simulink model "main_simulink"  (R2019b)
settings: Solver=FixedStepAuto  StartTime=0.0  StopTime=2.5  FixedStep=0.01  RelTol=1e-3
values from neighbouring files (symbols this model uses):
  b = 0.1    [main.m]
  g = 9.8    [main.m]
  I = 0.006    [main.m]
  l = 0.3    [main.m]
  m = length(x)    [PRBS.m]    (also in gaplotbestindivg.m = sum(x) ./ n; main.m = 0.2)
  M = 0.5    [main.m]
libraries: simulink x1
settings Model: Creator=sansh  LastModifiedBy=rifky
settings DataIOCC: ReturnWorkspaceOutputs=off
settings DebuggingCC: ArithmeticOperatorsInVariantConditions=warning
settings SFSimCC: SimUseLocalCustomCode=off  CustomCodeUndefinedFunction=UseInterfaceOnly
settings RTWCC: RTWUseLocalCustomCode=off
settings CodeAppCC: StateflowObjectComments=on

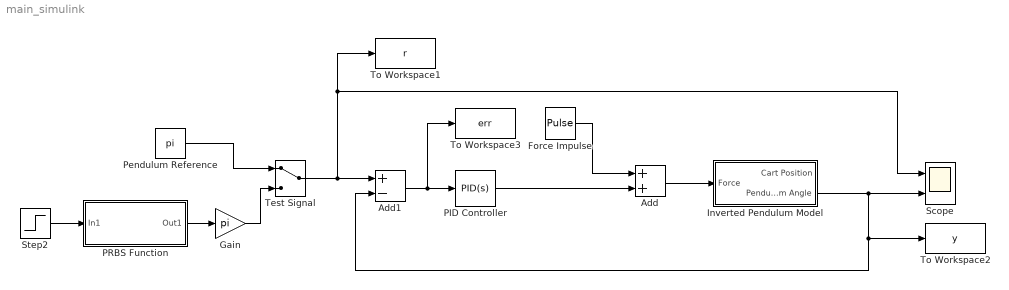
== system main_simulink ==
  Add : Sum
  Add1 : Sum  Inputs=+-
  Force Impulse : DiscretePulseGenerator  PulseType=Time based  Amplitude=1000  Period=10  PulseWidth=0.1
  Gain : Gain  Gain=pi
  Inverted Pendulum Model : Subsystem
  PID Controller : simulink/Continuous/PID Controller  Controller=PID  Form=Parallel  TimeDomain=Continuous-time  SampleTime=-1  IntegratorMethod=Forward Euler  FilterMethod=Forward Euler  ControllerParametersSource=internal  P=csvread('kp.dat')  I=csvread('ki.dat')  D=csvread('kd.dat')  UseFilter=on  N=100  TunerSelectOption=Transfer Function Based (PID Tuner App)  InitialConditionSource=internal  InitialConditionForIntegrator=0  InitialConditionForFilter=0  DifferentiatorICPrevScaledInput=0  ExternalReset=none  TrackingMode=off  Kt=1  LimitOutput=off  UpperSaturationLimit=inf  LowerSaturationLimit=-inf  LinearizeAsGain=on  AntiWindupMode=none  Kb=1  POutMin=[]  POutMax=[]  IOutMin=[]  IOutMax=[]  DOutMin=[]  DOutMax=[]  NOutMin=[]  NOutMax=[]  SumOutMin=[]  SumOutMax=[]  SaturationOutMin=[]  SaturationOutMax=[]  PParamMin=[]  PParamMax=[]  IParamMin=[]  IParamMax=[]  DParamMin=[]  DParamMax=[]  NParamMin=[]  NParamMax=[]  KbParamMin=[]  KbParamMax=[]  KtParamMin=[]  KtParamMax=[]  KbOutMin=[]  KbOutMax=[]  KtOutMin=[]  KtOutMax=[]  IntegratorOutMin=[]  IntegratorOutMax=[]  FilterOutMin=[]  FilterOutMax=[]  SumI1OutMin=[]  SumI1OutMax=[]  SumI2OutMin=[]  SumI2OutMax=[]  SumI3OutMin=[]  SumI3OutMax=[]  SumI4OutMin=[]  SumI4OutMax=[]  SumDOutMin=[]  SumDOutMax=[]  DifferentiatorOutMin=[]  DifferentiatorOutMax=[]  FilterDiffOutCoefMin=[]  FilterDiffOutCoefMax=[]  ReciprocalOutMin=[]  ReciprocalOutMax=[]  SumDenOutMin=[]  SumDenOutMax=[]  SumNumOutMin=[]  SumNumOutMax=[]  DivideOutMin=[]  DivideOutMax=[]  IntegratorContinuousStateAttributes=''  IntegratorStateMustResolveToSignalObject=off  IntegratorRTWStateStorageClass=Auto  FilterContinuousStateAttributes=''  FilterStateMustResolveToSignalObject=off  FilterRTWStateStorageClass=Auto  ParallelPVariant=InternalParameters  IdealPVariant=Disabled  IVariant=InternalParameters  DVariant=InternalParameters  IntegratorVariant=Continuous  SatVariant=Disabled  AWVariant=Passthrough  PCopyVariant=Disabled  TRVariant=Disabled  FdbkBlocksVariant=Forward  IdealPFdbkVariant=Disabled  SatFdbkVariant=Disabled  DerivativeFilterVariant=ContFilter  NVariant=InternalParameters  NCopyVariant=Disabled  FilterICVariant=InternalICsFilter  IntegratorICVariant=InternalICs  ExternalResetVariant=Disabled  TRSumVariant=Passthrough  SumFdbkVariant=Disabled  SumVariant=Sum_PID
  PRBS Function : Subsystem
  Pendulum Reference : Constant  Value=pi
  Scope : Scope  NumInputPorts=2
  Step2 : Step  After=0  SampleTime=0
  Test Signal : ManualSwitch
  To Workspace1 : ToWorkspace  VariableName=r  SampleTime=-1
  To Workspace2 : ToWorkspace  VariableName=y  SampleTime=-1
  To Workspace3 : ToWorkspace  VariableName=err  SaveFormat=Structure With Time  SampleTime=-1
  wires:
  Add1/1 -> To Workspace3/1, PID Controller/1
  PID Controller/1 -> Add/2
  Force Impulse/1 -> Add/1
  Add/1 -> Inverted Pendulum Model/1(Force)
  Inverted Pendulum Model/2(Pendulum Angle) -> To Workspace2/1, Add1/2, Scope/2
  Step2/1 -> PRBS Function/1(In1)
  Pendulum Reference/1 -> Test Signal/1
  PRBS Function/1(Out1) -> Gain/1
  Gain/1 -> Test Signal/2
  Test Signal/1 -> To Workspace1/1, Scope/1, Add1/1

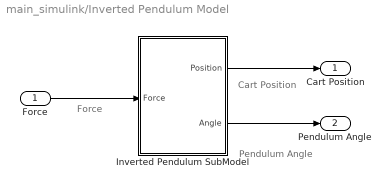
== system main_simulink/Inverted Pendulum Model ==
  note: Force
  note: Pendulum Angle
  note: Cart Position
  Force : Inport
  Inverted Pendulum SubModel : Subsystem
  Cart Position : Outport
  Pendulum Angle : Outport  Port=2
  wires:
  Inverted Pendulum SubModel/2(Angle) -> Pendulum Angle/1
  Inverted Pendulum SubModel/1(Position) -> Cart Position/1
  Force/1 -> Inverted Pendulum SubModel/1(Force)

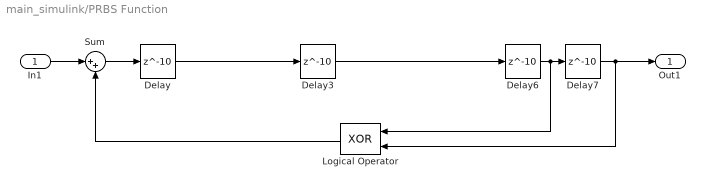
== system main_simulink/PRBS Function ==
  In1 : Inport
  Delay : Delay  DelayLength=10  InitialCondition=0
  Delay3 : Delay  DelayLength=10
  Delay6 : Delay  DelayLength=10
  Delay7 : Delay  DelayLength=10  InitialCondition=1
  Logical Operator : Logic  Operator=XOR  AllPortsSameDT=off  OutDataTypeStr=boolean
  Sum : Sum  Inputs=|++
  Out1 : Outport
  wires:
  Delay6/1 -> Logical Operator/1, Delay7/1
  Delay7/1 -> Out1/1, Logical Operator/2
  Sum/1 -> Delay/1
  Logical Operator/1 -> Sum/2
  In1/1 -> Sum/1
  Delay/1 -> Delay3/1
  Delay3/1 -> Delay6/1

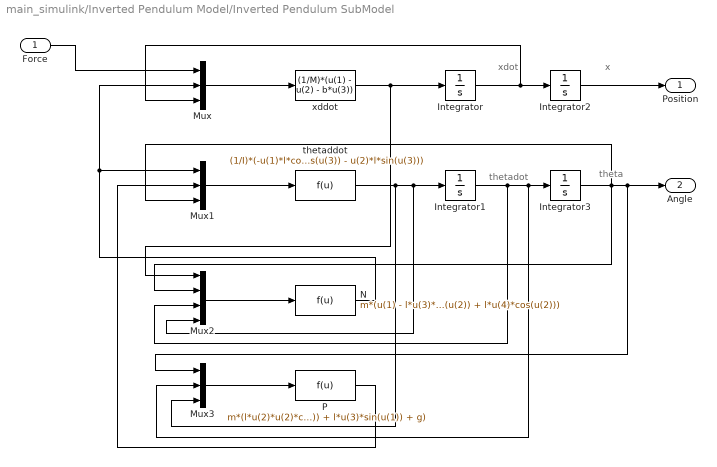
== system main_simulink/Inverted Pendulum Model/Inverted Pendulum SubModel ==
  note: theta
  note: x
  note: thetadot
  note: xdot
  Force : Inport
  Integrator : Integrator  ContinuousStateAttributes='xdot'
  Integrator1 : Integrator  ContinuousStateAttributes='thetadot'
  Integrator2 : Integrator  ContinuousStateAttributes='x'
  Integrator3 : Integrator  InitialCondition=-pi  ContinuousStateAttributes='theta'
  Mux : Mux  Inputs=3
  Mux1 : Mux  Inputs=3
  Mux2 : Mux
  Mux3 : Mux  Inputs=3
  N : Fcn  Expr=m*(u(1) - l*u(3)*u(3)*sin(u(2)) + l*u(4)*cos(u(2)))
  P : Fcn  Expr=m*(l*u(2)*u(2)*cos(u(1)) + l*u(3)*sin(u(1)) + g)
  thetaddot : Fcn  Expr=(1/I)*(-u(1)*l*cos(u(3)) - u(2)*l*sin(u(3)))
  xddot : Fcn  Expr=(1/M)*(u(1) - u(2) - b*u(3))
  Position : Outport
  Angle : Outport  Port=2
  wires:
  Force/1 -> Mux/1
  Mux2/1 -> N/1
  Mux/1 -> xddot/1
  P/1 -> Mux1/2
  Mux3/1 -> P/1
  N/1 -> Mux1/1, Mux/2
  Mux1/1 -> thetaddot/1
  xddot/1 -> Mux2/1, Integrator/1
  Integrator2/1 -> Position/1
  thetaddot/1 -> Mux3/3, Mux2/4, Integrator1/1
  Integrator/1 -> Mux/3, Integrator2/1
  Integrator1/1 -> Mux2/3, Mux3/2, Integrator3/1
  Integrator3/1 -> Mux2/2, Mux1/3, Angle/1, Mux3/1
